simulink model "EAF_simscape"  (R2025b)
settings: Solver=ode23t  StartTime=0.0  StopTime=5  RelTol=1e-3
undefined symbols (not defined in the file or in its folder): Three_PhaseSeriesRLCLoad_class, Three_PhaseSource_class, Three_PhaseTransformer_2_class, Three_PhaseTransformer_T_class, Three_PhaseV_IMeasuremen_class
libraries: ee_lib x12, nesl_utility x9, fl_lib x6, elec_conv_Three_PhaseV_IMeasuremen x4, eeRmsMeasurement x3, elec_conv_sl_RMS x3, spsVariableResistorLib x3, elec_conv_Three_PhaseSeriesRLCBran x3, elec_conv_Three_PhaseSeriesRLCLoad x2, elec_conv_Three_PhaseTransformer_2 x2, elec_conv_Three_PhaseTransformer_T x1, elec_conv_Three_PhaseSource x1
(part 1 of 2)
settings Model: Creator=LYG  LastModifiedBy=LYG
settings DebuggingCC: SaveWithParameterizedLinksMsg=none

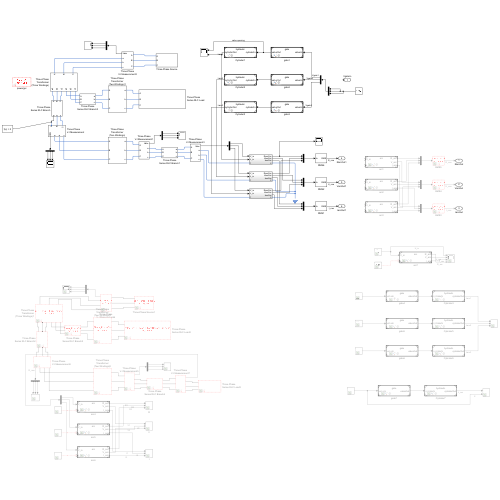
[thumbnail: Simulink's stored preview of the top-level diagram]
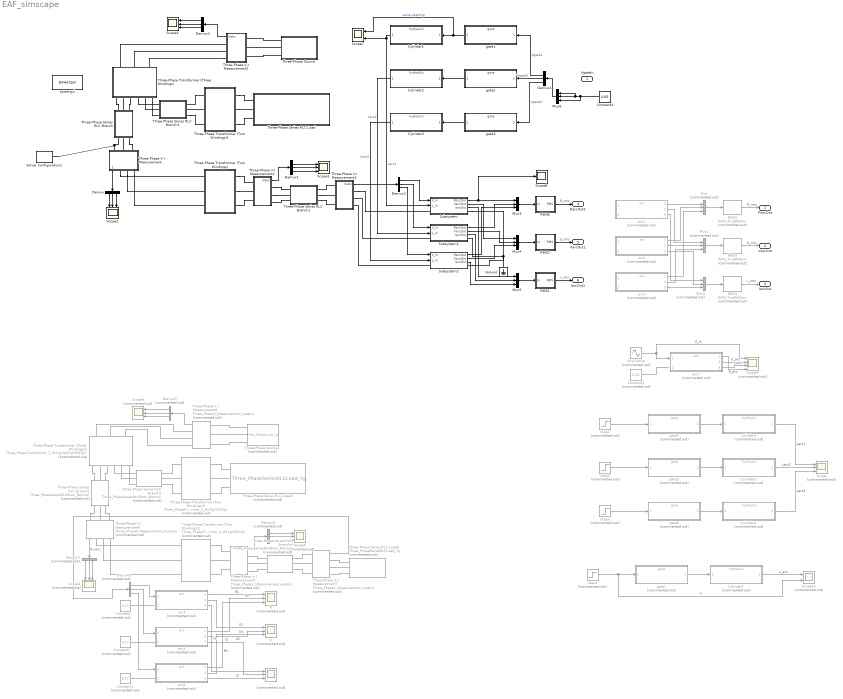
== system EAF_simscape ==
  VgateIn : Inport
  Constant : Constant  Commented=on  Value=0.17
  Constant1 : Constant  Commented=on  Value=0.17
  Constant2 : Constant  Commented=on  Value=0.17
  Constant3 : Constant  Commented=on  Value=0.15
  Constant4 : Constant  Value=0.65
  Cylinder1 : ModelReference  ModelNameDialog=hydraulic.slx  UsingDefaultArgumentValue=0,0,0,0,0,0,0,0,0  SimulationMode=Normal  ModelReferenceVersion=1.17  Ap=0.0314  Ct=2.4e-12  Fforce=90000  Gmass=9000  Kc=1.68e-9  Kq=1.63  Ve=0.11304  beta_e=7e8  L_init=0.15
  Cylinder2 : ModelReference  ModelNameDialog=hydraulic.slx  UsingDefaultArgumentValue=0,0,0,0,0,0,0,0,0  SimulationMode=Normal  ModelReferenceVersion=1.17  Ap=0.0314  Ct=2.4e-12  Fforce=90000  Gmass=9000  Kc=1.68e-9  Kq=1.63  Ve=0.11304  beta_e=7e8  L_init=0.15
  Cylinder3 : ModelReference  ModelNameDialog=hydraulic.slx  UsingDefaultArgumentValue=0,0,0,0,0,0,0,0,0  SimulationMode=Normal  ModelReferenceVersion=1.17  Ap=0.0314  Ct=2.4e-12  Fforce=90000  Gmass=9000  Kc=1.68e-9  Kq=1.63  Ve=0.11304  beta_e=7e8  L_init=0.15
  Cylinder4 : ModelReference  Commented=on  ModelNameDialog=hydraulic.slx  UsingDefaultArgumentValue=0,0,0,0,0,0,0,0,0  SimulationMode=Normal  ModelReferenceVersion=1.17  Ap=0.0314  Ct=2.4e-12  Fforce=90000  Gmass=9000  Kc=1.68e-9  Kq=1.63  Ve=0.11304  beta_e=7e8  L_init=15
  Cylinder5 : ModelReference  Commented=on  ModelNameDialog=hydraulic.slx  UsingDefaultArgumentValue=0,0,0,0,0,0,0,0,0  SimulationMode=Normal  ModelReferenceVersion=1.17  Ap=0.0314  Ct=2.4e-12  Fforce=90000  Gmass=9000  Kc=1.68e-9  Kq=1.63  Ve=0.11304  beta_e=7e8  L_init=15
  Cylinder6 : ModelReference  Commented=on  ModelNameDialog=hydraulic.slx  UsingDefaultArgumentValue=0,0,0,0,0,0,0,0,0  SimulationMode=Normal  ModelReferenceVersion=1.17  Ap=0.0314  Ct=2.4e-12  Fforce=90000  Gmass=9000  Kc=1.68e-9  Kq=1.63  Ve=0.11304  beta_e=7e8  L_init=15
  Cylinder7 : ModelReference  Commented=on  ModelNameDialog=hydraulic.slx  UsingDefaultArgumentValue=0,0,0,0,0,0,0,0,0  SimulationMode=Normal  ModelReferenceVersion=1.17  Ap=0.0314  Ct=2.4e-12  Fforce=90000  Gmass=9000  Kc=1.68e-9  Kq=1.63  Ve=0.11304  beta_e=7e8  L_init=0.5
  Demux{,1..4} (5 alike) : Demux  Outputs=3
  Demux{5..8} (4 alike) : Demux  Commented=on  Outputs=3
  Ground : fl_lib/Electrical/Electrical Elements/Electrical Reference
  I : Scope  Commented=on  NumInputPorts=3
      settings: ActiveDisplayYMinimum=-181487.67004  ActiveDisplayYMaximum=204820.87282  DataLoggingVariableName=ScopeData4
  Mux : Mux  Commented=on  Inputs=3
  Mux1 : Mux  Commented=on  Inputs=3
  Mux2 : Mux  Commented=on  Inputs=3
  Mux{3..6} (4 alike) : Mux  Inputs=3
  R : Scope  Commented=on  NumInputPorts=3
      settings: ActiveDisplayYMinimum=-0.00531  ActiveDisplayYMaximum=0.04981  DataLoggingVariableName=ScopeData5
  RMS1 : Subsystem
      settings: OpenFcn=elec.conv.unmask(gcb);
  RMS2 : Subsystem
      settings: OpenFcn=elec.conv.unmask(gcb);
  RMS3 : elec_conv_sl_RMS/RMS_TrueRMSon  Commented=on  SystemSampleTime=-1  VariantActivationTime=update diagram  EmptyChoice=off  PassThrough=off  PassThroughVariantControl=(default)  EmptyChoiceVariantControl=(default)  AllowFlexibleInterface=on  Latency=0  AutoFrameSizeCalculation=off
  RMS4 : elec_conv_sl_RMS/RMS_TrueRMSon  Commented=on  SystemSampleTime=-1  VariantActivationTime=update diagram  EmptyChoice=off  PassThrough=off  PassThroughVariantControl=(default)  EmptyChoiceVariantControl=(default)  AllowFlexibleInterface=on  Latency=0  AutoFrameSizeCalculation=off
  RMS5 : elec_conv_sl_RMS/RMS_TrueRMSon  Commented=on  SystemSampleTime=-1  VariantActivationTime=update diagram  EmptyChoice=off  PassThrough=off  PassThroughVariantControl=(default)  EmptyChoiceVariantControl=(default)  AllowFlexibleInterface=on  Latency=0  AutoFrameSizeCalculation=off
  RMS6 : Subsystem
      settings: OpenFcn=elec.conv.unmask(gcb);
  Scope{,1,5..6} (4 alike) : Scope  Commented=on  NumInputPorts=3
      Scope settings: ActiveDisplayYMinimum=13.76369  ActiveDisplayYMaximum=16.01617  DataLoggingVariableName=ScopeData4
      Scope1 settings: ActiveDisplayYMinimum=-4346.80314  ActiveDisplayYMaximum=39121.22823
      Scope5 settings: ActiveDisplayYMinimum=-7403.31219  ActiveDisplayYMaximum=7403.31279  DataLoggingVariableName=ScopeData2
      Scope6 settings: ActiveDisplayYMinimum=-194335.71856  ActiveDisplayYMaximum=194335.71856  DataLoggingVariableName=ScopeData3
  Scope10 : Scope  Commented=on  NumInputPorts=2
      settings: ActiveDisplayYMinimum=0.16708  ActiveDisplayYMaximum=1.06427  DataLoggingVariableName=ScopeData2
  Scope2 : Scope  NumInputPorts=3
      settings: ActiveDisplayYMinimum=-54351.26141  ActiveDisplayYMaximum=61130.65536
  Scope3 : Scope  NumInputPorts=3
      settings: ActiveDisplayYMinimum=-666.22173  ActiveDisplayYMaximum=595.66342  DataLoggingVariableName=ScopeData2
  Scope4 : Scope  NumInputPorts=3
      settings: ActiveDisplayYMinimum=-194453.93834  ActiveDisplayYMaximum=194453.93834  DataLoggingVariableName=ScopeData3
  Scope7 : Scope  NumInputPorts=2
      settings: ActiveDisplayYMinimum=-0.00342  ActiveDisplayYMaximum=0.00705
  Scope8 : Scope
      settings: ActiveDisplayYMinimum=-66.36555  ActiveDisplayYMaximum=597.29198
  Scope9 : Scope  Commented=on  NumInputPorts=4
      settings: ActiveDisplayYMinimum=-429.56648  ActiveDisplayYMaximum=429.56274
  Sine Wave : Sin  Commented=on  Amplitude=sqrt(2) * 243  Frequency=2 * pi * 60  SampleTime=0
  Solver Configuration1 : nesl_utility/Solver Configuration  PhysicalDomain=network_engine_domain  SubClassName=solver  LeftPortType=input  RightPortType=generic  Tones=[]  Harmonics=[]  SimulateNoise=off  Profile=off  UseLocalSampling=off  EnableSwitchedLinearOptims=on  FrequencyDomain=off  UseCCode=off  RelTol=0.001  AbsTol=0.001  MinStep=1e-09  ToWorkspace=off  RevertToSquareIcSolve=off  NumHomotopyIterations=100  PhasorMode=off  PhasorModeNumHarmonics=1  ConsistencySolver=NEWTON_XTOL_AFTER_FTOL  IndexReductionMethod=DerivativeReplacement  DoDC=off  ResidualTolerance=1e-09  ConsistencyTolSource=GLOBAL  ConsistencyAbsTol=0.001  ConsistencyRelTol=0.001  ConsistencyTolFactor=0.001  UseLocalSolver=off  LocalSolverChoice=NE_BACKWARD_EULER_ADVANCER  ResolveIndetEquations=on  FunctionEvalNumThread=1  LocalSolverSampleTime=0.001  DoFixedCost=off  MaxNonlinIter=3  MaxModeIter=2  ComputeImpulses=off  ImpulseIterations=2  LinearAlgebra=auto  LinearAlgebraNumThread=0  EquationFormulation=NE_TIME_EF  DelaysMemoryBudget=1024  AutomaticFiltering=on  FilteringTimeConstant=0.001  PartitionStorageMethod=AS_NEEDED  PartitionMemoryBudget=1024  PartitionMethod=ROBUST  MultibodyUseLocalSolver=off  MultibodyLocalSolverChoice=ODE1  MultibodyLocalSolverSampleTime=0.001
  Step1 : Step  Commented=on  Time=5  After=5  SampleTime=0
  Step2 : Step  Commented=on  Time=5  Before=5  After=0  SampleTime=0
  Step3 : Step  Commented=on  Time=3  Before=5  After=-5  SampleTime=0
  Step4 : Step  Commented=on  Time=3  Before=5  After=-5  SampleTime=0
  Subsystem : Subsystem
  Subsystem1 : Subsystem
  Subsystem2 : Subsystem
  Three-Phase Series RLC Branch : Subsystem
      settings: AttributesFormatString=\n  OpenFcn=elec.conv.unmask(gcb);
  Three-Phase Series RLC Branch1 : Subsystem
      settings: AttributesFormatString=\n  OpenFcn=elec.conv.unmask(gcb);
  Three-Phase Series RLC Branch2 : elec_conv_Three_PhaseSeriesRLCBran/Three_PhaseSeriesRLCBran_Normal  Commented=on  component_structure=1  R=0.256  L=0.001  C=1e-06
      settings: AttributesFormatString=\n
  Three-Phase Series RLC Branch3 : Subsystem
      settings: AttributesFormatString=\n  OpenFcn=elec.conv.unmask(gcb);
  Three-Phase Series RLC Branch4 : elec_conv_Three_PhaseSeriesRLCBran/Three_PhaseSeriesRLCBran_Normal  Commented=on  component_structure=4  R=0.0004  L=1.115e-05  C=1e-06
      settings: AttributesFormatString=\n
  Three-Phase Series RLC Branch5 : elec_conv_Three_PhaseSeriesRLCBran/Three_PhaseSeriesRLCBran_Normal  Commented=on  component_structure=1  R=0.256  L=0.001  C=1e-06
      settings: AttributesFormatString=\n
  Three-Phase Series RLC Load : Subsystem
      settings: AttributesFormatString=\n  OpenFcn=elec.conv.unmask(gcb);
  Three-Phase Series RLC Load2 : elec_conv_Three_PhaseSeriesRLCLoad/Three_PhaseSeriesRLCLoad_Yg  Commented=on  VRated=1000  Vmag0=1000  FRated=60  P=10000  Qpos=100  Qneg=Three_PhaseSeriesRLCLoad_class(100).objParamMappingDerived.NewDerivedParam.Qneg  component_structure_PQ=7  component_structure=7
      settings: AttributesFormatString=\n
  Three-Phase Series RLC Load3 : elec_conv_Three_PhaseSeriesRLCLoad/Three_PhaseSeriesRLCLoad_Yg  Commented=on  VRated=1000  Vmag0=1000  FRated=60  P=10000  Qpos=100  Qneg=Three_PhaseSeriesRLCLoad_class(100).objParamMappingDerived.NewDerivedParam.Qneg  component_structure_PQ=7  component_structure=7
      settings: AttributesFormatString=\n
  Three-Phase Transformer (Three Windings) : Subsystem
      settings: OpenFcn=elec.conv.unmask(gcb);
  Three-Phase Transformer (Three Windings)1 : elec_conv_Three_PhaseTransformer_T/Three_PhaseTransformer_T_W1YgYW2YgYW3YgY  Commented=on  SRated=250000000  FRated=60  VRated1=110000  VRated2=35000  VRated3=35000  phi_specify=off  phi_priority=None  pu_Rw1=Three_PhaseTransformer_T_class('Yg','Yg','Yg','pu',[250000000 60],[110000 1.186 0.08],[35000 0.256 0.08],[35000 0.002 0.08],499.98,500,0.5,[0 0;0.0024 1.2;1 1.52],[0.8 -0.8 0.69999],'off','off').objParamMappingDerived.NewDerivedParam.pu_Rw1  pu_Xl1=Three_PhaseTransformer_T_class('Yg','Yg','Yg','pu',[250000000 60],[110000 1.186 0.08],[35000 0.256 0.08],[35000 0.002 0.08],499.98,500,0.5,[0 0;0.0024 1.2;1 1.52],[0.8 -0.8 0.69999],'off','off').objParamMappingDerived.NewDerivedParam.pu_Xl1  pu_Rw2=Three_PhaseTransformer_T_class('Yg','Yg','Yg','pu',[250000000 60],[110000 1.186 0.08],[35000 0.256 0.08],[35000 0.002 0.08],499.98,500,0.5,[0 0;0.0024 1.2;1 1.52],[0.8 -0.8 0.69999],'off','off').objParamMappingDerived.NewDerivedParam.pu_Rw2  pu_Xl2=Three_PhaseTransformer_T_class('Yg','Yg','Yg','pu',[250000000 60],[110000 1.186 0.08],[35000 0.256 0.08],[35000 0.002 0.08],499.98,500,0.5,[0 0;0.0024 1.2;1 1.52],[0.8 -0.8 0.69999],'off','off').objParamMappingDerived.NewDerivedParam.pu_Xl2  pu_Rw3=Three_PhaseTransformer_T_class('Yg','Yg','Yg','pu',[250000000 60],[110000 1.186 0.08],[35000 0.256 0.08],[35000 0.002 0.08],499.98,500,0.5,[0 0;0.0024 1.2;1 1.52],[0.8 -0.8 0.69999],'off','off').objParamMappingDerived.NewDerivedParam.pu_Rw3  pu_Xl3=Three_PhaseTransformer_T_class('Yg','Yg','Yg','pu',[250000000 60],[110000 1.186 0.08],[35000 0.256 0.08],[35000 0.002 0.08],499.98,500,0.5,[0 0;0.0024 1.2;1 1.52],[0.8 -0.8 0.69999],'off','off').objParamMappingDerived.NewDerivedParam.pu_Xl3  pu_Rm=Three_PhaseTransformer_T_class('Yg','Yg','Yg','pu',[250000000 60],[110000 1.186 0.08],[35000 0.256 0.08],[35000 0.002 0.08],499.98,500,0.5,[0 0;0.0024 1.2;1 1.52],[0.8 -0.8 0.69999],'off','off').objParamMappingDerived.NewDerivedParam.pu_Rm  pu_Xm=Three_PhaseTransformer_T_class('Yg','Yg','Yg','pu',[250000000 60],[110000 1.186 0.08],[35000 0.256 0.08],[35000 0.002 0.08],499.98,500,0.5,[0 0;0.0024 1.2;1 1.52],[0.8 -0.8 0.69999],'off','off').objParamMappingDerived.NewDerivedParam.pu_Xm  pu_X0=Three_PhaseTransformer_T_class('Yg','Yg','Yg','pu',[250000000 60],[110000 1.186 0.08],[35000 0.256 0.08],[35000 0.002 0.08],499.98,500,0.5,[0 0;0.0024 1.2;1 1.52],[0.8 -0.8 0.69999],'off','off').objParamMappingDerived.NewDerivedParam.pu_X0  current_data=Three_PhaseTransformer_T_class('Yg','Yg','Yg','pu',[250000000 60],[110000 1.186 0.08],[35000 0.256 0.08],[35000 0.002 0.08],499.98,500,0.5,[0 0;0.0024 1.2;1 1.52],[0.8 -0.8 0.69999],'off','off').objParamMappingDerived.NewDerivedParam.current_data  magnetic_flux_data=Three_PhaseTransformer_T_class('Yg','Yg','Yg','pu',[250000000 60],[110000 1.186 0.08],[35000 0.256 0.08],[35000 0.002 0.08],499.98,500,0.5,[0 0;0.0024 1.2;1 1.52],[0.8 -0.8 0.69999],'off','off').objParamMappingDerived.NewDerivedParam.magnetic_flux_data  phi=Three_PhaseTransformer_T_class('Yg','Yg','Yg','pu',[250000000 60],[110000 1.186 0.08],[35000 0.256 0.08],[35000 0.002 0.08],499.98,500,0.5,[0 0;0.0024 1.2;1 1.52],[0.8 -0.8 0.69999],'off','off').objParamMappingDerived.NewDerivedParam.phi  Winding1Connection=3  Winding2Connection=3  Winding3Connection=3  saturation_option=1  CoreType=2
  Three-Phase Transformer (Two Windings) : Subsystem
      settings: OpenFcn=elec.conv.unmask(gcb);
  Three-Phase Transformer (Two Windings)1 : Subsystem
      settings: OpenFcn=elec.conv.unmask(gcb);
  Three-Phase Transformer (Two Windings)2 : elec_conv_Three_PhaseTransformer_2/Three_PhaseTransformer_2_W1YgYW2YgY  Commented=on  SRated=250000000  FRated=60  VRated1=35000  VRated2=440.02  phi_specify=off  phi_priority=None  pu_Rw1=Three_PhaseTransformer_2_class('Yg','Yg','pu',[250000000 60],[35000 6.9e-05 2.2e-06],[440.02 6.9e-05 2.2e-06],500,500,0.5,[0 0;0.0024 1.2;1 1.52],[0.8 -0.8 0.7],'off','off').objParamMappingDerived.NewDerivedParam.pu_Rw1  pu_Xl1=Three_PhaseTransformer_2_class('Yg','Yg','pu',[250000000 60],[35000 6.9e-05 2.2e-06],[440.02 6.9e-05 2.2e-06],500,500,0.5,[0 0;0.0024 1.2;1 1.52],[0.8 -0.8 0.7],'off','off').objParamMappingDerived.NewDerivedParam.pu_Xl1  pu_Rw2=Three_PhaseTransformer_2_class('Yg','Yg','pu',[250000000 60],[35000 6.9e-05 2.2e-06],[440.02 6.9e-05 2.2e-06],500,500,0.5,[0 0;0.0024 1.2;1 1.52],[0.8 -0.8 0.7],'off','off').objParamMappingDerived.NewDerivedParam.pu_Rw2  pu_Xl2=Three_PhaseTransformer_2_class('Yg','Yg','pu',[250000000 60],[35000 6.9e-05 2.2e-06],[440.02 6.9e-05 2.2e-06],500,500,0.5,[0 0;0.0024 1.2;1 1.52],[0.8 -0.8 0.7],'off','off').objParamMappingDerived.NewDerivedParam.pu_Xl2  pu_Rm=Three_PhaseTransformer_2_class('Yg','Yg','pu',[250000000 60],[35000 6.9e-05 2.2e-06],[440.02 6.9e-05 2.2e-06],500,500,0.5,[0 0;0.0024 1.2;1 1.52],[0.8 -0.8 0.7],'off','off').objParamMappingDerived.NewDerivedParam.pu_Rm  pu_Xm=Three_PhaseTransformer_2_class('Yg','Yg','pu',[250000000 60],[35000 6.9e-05 2.2e-06],[440.02 6.9e-05 2.2e-06],500,500,0.5,[0 0;0.0024 1.2;1 1.52],[0.8 -0.8 0.7],'off','off').objParamMappingDerived.NewDerivedParam.pu_Xm  pu_X0=Three_PhaseTransformer_2_class('Yg','Yg','pu',[250000000 60],[35000 6.9e-05 2.2e-06],[440.02 6.9e-05 2.2e-06],500,500,0.5,[0 0;0.0024 1.2;1 1.52],[0.8 -0.8 0.7],'off','off').objParamMappingDerived.NewDerivedParam.pu_X0  current_data=Three_PhaseTransformer_2_class('Yg','Yg','pu',[250000000 60],[35000 6.9e-05 2.2e-06],[440.02 6.9e-05 2.2e-06],500,500,0.5,[0 0;0.0024 1.2;1 1.52],[0.8 -0.8 0.7],'off','off').objParamMappingDerived.NewDerivedParam.current_data  magnetic_flux_data=Three_PhaseTransformer_2_class('Yg','Yg','pu',[250000000 60],[35000 6.9e-05 2.2e-06],[440.02 6.9e-05 2.2e-06],500,500,0.5,[0 0;0.0024 1.2;1 1.52],[0.8 -0.8 0.7],'off','off').objParamMappingDerived.NewDerivedParam.magnetic_flux_data  phi=Three_PhaseTransformer_2_class('Yg','Yg','pu',[250000000 60],[35000 6.9e-05 2.2e-06],[440.02 6.9e-05 2.2e-06],500,500,0.5,[0 0;0.0024 1.2;1 1.52],[0.8 -0.8 0.7],'off','off').objParamMappingDerived.NewDerivedParam.phi  Winding1Connection=3  Winding2Connection=3  saturation_option=1  CoreType=2
  Three-Phase Transformer (Two Windings)3 : elec_conv_Three_PhaseTransformer_2/Three_PhaseTransformer_2_W1YgYW2YgY  Commented=on  SRated=250000000  FRated=60  VRated1=735000  VRated2=8820  phi_specify=off  phi_priority=None  pu_Rw1=Three_PhaseTransformer_2_class('Yg','Yg','pu',[250000000 60],[735000 6.9e-05 2.2e-06],[8820 6.9e-05 2.2e-06],500,500,0.5,[0 0;0.0024 1.2;1 1.52],[0.8 -0.8 0.7],'off','off').objParamMappingDerived.NewDerivedParam.pu_Rw1  pu_Xl1=Three_PhaseTransformer_2_class('Yg','Yg','pu',[250000000 60],[735000 6.9e-05 2.2e-06],[8820 6.9e-05 2.2e-06],500,500,0.5,[0 0;0.0024 1.2;1 1.52],[0.8 -0.8 0.7],'off','off').objParamMappingDerived.NewDerivedParam.pu_Xl1  pu_Rw2=Three_PhaseTransformer_2_class('Yg','Yg','pu',[250000000 60],[735000 6.9e-05 2.2e-06],[8820 6.9e-05 2.2e-06],500,500,0.5,[0 0;0.0024 1.2;1 1.52],[0.8 -0.8 0.7],'off','off').objParamMappingDerived.NewDerivedParam.pu_Rw2  pu_Xl2=Three_PhaseTransformer_2_class('Yg','Yg','pu',[250000000 60],[735000 6.9e-05 2.2e-06],[8820 6.9e-05 2.2e-06],500,500,0.5,[0 0;0.0024 1.2;1 1.52],[0.8 -0.8 0.7],'off','off').objParamMappingDerived.NewDerivedParam.pu_Xl2  pu_Rm=Three_PhaseTransformer_2_class('Yg','Yg','pu',[250000000 60],[735000 6.9e-05 2.2e-06],[8820 6.9e-05 2.2e-06],500,500,0.5,[0 0;0.0024 1.2;1 1.52],[0.8 -0.8 0.7],'off','off').objParamMappingDerived.NewDerivedParam.pu_Rm  pu_Xm=Three_PhaseTransformer_2_class('Yg','Yg','pu',[250000000 60],[735000 6.9e-05 2.2e-06],[8820 6.9e-05 2.2e-06],500,500,0.5,[0 0;0.0024 1.2;1 1.52],[0.8 -0.8 0.7],'off','off').objParamMappingDerived.NewDerivedParam.pu_Xm  pu_X0=Three_PhaseTransformer_2_class('Yg','Yg','pu',[250000000 60],[735000 6.9e-05 2.2e-06],[8820 6.9e-05 2.2e-06],500,500,0.5,[0 0;0.0024 1.2;1 1.52],[0.8 -0.8 0.7],'off','off').objParamMappingDerived.NewDerivedParam.pu_X0  current_data=Three_PhaseTransformer_2_class('Yg','Yg','pu',[250000000 60],[735000 6.9e-05 2.2e-06],[8820 6.9e-05 2.2e-06],500,500,0.5,[0 0;0.0024 1.2;1 1.52],[0.8 -0.8 0.7],'off','off').objParamMappingDerived.NewDerivedParam.current_data  magnetic_flux_data=Three_PhaseTransformer_2_class('Yg','Yg','pu',[250000000 60],[735000 6.9e-05 2.2e-06],[8820 6.9e-05 2.2e-06],500,500,0.5,[0 0;0.0024 1.2;1 1.52],[0.8 -0.8 0.7],'off','off').objParamMappingDerived.NewDerivedParam.magnetic_flux_data  phi=Three_PhaseTransformer_2_class('Yg','Yg','pu',[250000000 60],[735000 6.9e-05 2.2e-06],[8820 6.9e-05 2.2e-06],500,500,0.5,[0 0;0.0024 1.2;1 1.52],[0.8 -0.8 0.7],'off','off').objParamMappingDerived.NewDerivedParam.phi  Winding1Connection=3  Winding2Connection=3  saturation_option=1  CoreType=2
  Three-Phase V-I Measurement : Subsystem
      settings: OpenFcn=elec.conv.unmask(gcb);
  Three-Phase V-I Measurement1 : Subsystem
      settings: OpenFcn=elec.conv.unmask(gcb);
  Three-Phase V-I Measurement2 : Subsystem
      settings: OpenFcn=elec.conv.unmask(gcb);
  Three-Phase V-I Measurement3 : Subsystem
      settings: OpenFcn=elec.conv.unmask(gcb);
  Three-Phase V-I Measurement{4..7} (4 alike) : elec_conv_Three_PhaseV_IMeasuremen/Three_PhaseV_IMeasuremen_VyesIno  Commented=on  SRated=100000000  VRated=500000  vMeasurementType=1  outputUnit=2  GotoTagI=Iabc  GotoTagV=Vabc  IG=Three_PhaseV_IMeasuremen_class('phase-to-phase','no','off','off','off',100000000,500000).objParamMappingDerived.NewDerivedParam.IG  VG=Three_PhaseV_IMeasuremen_class('phase-to-phase','no','off','off','off',100000000,500000).objParamMappingDerived.NewDerivedParam.VG
  Three-Phase Source : Subsystem
      settings: OpenFcn=elec.conv.unmask(gcb);
  Three-Phase Source1 : elec_conv_Three_PhaseSource/Three_PhaseSource_Yg  Commented=on  vline_rms=110000  shift=0  freq=60  SShortCircuit=100000000  XR=7  R=Three_PhaseSource_class(110000,60,1.186,0.01658,100000000,110000,7,'on','off').objParamMappingDerived.NewDerivedParam.R  L=Three_PhaseSource_class(110000,60,1.186,0.01658,100000000,110000,7,'on','off').objParamMappingDerived.NewDerivedParam.L  impedance_option=4
  V : Scope  Commented=on  NumInputPorts=3
      settings: ActiveDisplayYMinimum=-330.37837  ActiveDisplayYMaximum=329.45455
  arc{1..7} (7 alike) : ModelReference  Commented=on  ModelNameDialog=arc.slx  UsingDefaultArgumentValue=0,0,0,0,0,0,0  SimulationMode=Normal  ModelReferenceVersion=1.20  K1=221320  K2=0.00072  lambda=2  Xd=3e-3  rd=0.4e-3  f=50  U_PhaseRMS=243
  gate1 : ModelReference  ModelNameDialog=gate.slx  UsingDefaultArgumentValue=0,0,0,0,0,0,0  SimulationMode=Normal  ModelReferenceVersion=1.12  Ksvr=0.04  Ksvl=0.0276  Xmax=0.006  Xmin=-0.004  dl=-0.014  dr=0.014  k=0.15
  gate2 : ModelReference  ModelNameDialog=gate.slx  UsingDefaultArgumentValue=0,0,0,0,0,0,0  SimulationMode=Normal  ModelReferenceVersion=1.12  Ksvr=0.04  Ksvl=0.0276  Xmax=0.006  Xmin=-0.004  dl=-0.014  dr=0.014  k=0.15
  gate3 : ModelReference  ModelNameDialog=gate.slx  UsingDefaultArgumentValue=0,0,0,0,0,0,0  SimulationMode=Normal  ModelReferenceVersion=1.12  Ksvr=0.04  Ksvl=0.0276  Xmax=0.006  Xmin=-0.004  dl=-0.014  dr=0.014  k=0.15
  gate{4..7} (4 alike) : ModelReference  Commented=on  ModelNameDialog=gate.slx  UsingDefaultArgumentValue=0,0,0,0,0,0,0  SimulationMode=Normal  ModelReferenceVersion=1.12  Ksvr=0.04  Ksvl=0.0276  Xmax=0.006  Xmin=-0.004  dl=-0.014  dr=0.014  k=0.15
  powergui : sps_lib/powergui  Priority=1  SimulationMode=Discrete  SampleTime=5e-5  frequency=60  Iterations=50  frequencyindice=60  Pbase=100e6  ErrMax=1e-4  UnitsV=kV  UnitsW=MW  buscounter=0  FunctionMessages=off  echomessages=off  EnableUseOfTLC=off  CurrentSourceSwitches=off  DisableSnubberDevices=off  DisableRonSwitches=off  DisableVfSwitches=off  DisplayEquations=off  AutomaticDiscreteSolvers=off  SolverType=Tustin/Backward Euler (TBE)  Interpol=off  ExternalGateDelay=off  methode=off  Ts=100  x0status=blocks  SPID=on  SwTol=0  HookPort=off  NonlinearTolerance=1e-4  nMaxIteration=100  ContinueOnMaxIteration=off  RestoreLinks=warning  ResistiveCurrentMeasurement=off  Frange=[0:2:500]  Ylog=off  Xlog=on  ShowGrid=off  save=off  variable=ZData  structure=0  ZoomFFT=off  StartTime=0.0  cycles=1  DisplayStyle=1  fundamental=60  FreqAxis=off  MaxFrequency=1000  frequencyindicesteady=1  RmsSteady=1  display=off
  RarcOut : Outport
  VarcOut : Outport  Port=2
  IarcOut : Outport  Port=3
  RarcOut1 : Outport  Port=4
  VarcOut1 : Outport  Port=5
  IarcOut1 : Outport  Port=6
  wires:
  Demux2/1 -> Scope4/1
  Demux2/3 -> Scope4/3
  Three-Phase V-I Measurement1/1(Vabc) -> Demux1/1
  Demux2/2 -> Scope4/2
  Demux1/3 -> Scope3/3
  Demux/2 -> Scope2/2
  Demux/1 -> Scope2/1
  Three-Phase V-I Measurement2/1(Vabc) -> Demux2/1
  Demux1/1 -> Scope3/1
  Three-Phase V-I Measurement/1(Vabc) -> Demux/1
  Demux/3 -> Scope2/3
  Demux1/2 -> Scope3/2
  gate2/1 -> Cylinder2/1
  gate1/1 -> Scope7/1, Cylinder1/1  "valve opening"
  gate3/1 -> Cylinder3/1
  Cylinder1/1 -> Subsystem/2(L_in), Scope7/2  "Larc1"
  Demux4/3 -> gate3/1  "Vgate3"
  Demux4/2 -> gate2/1  "Vgate2"
  Mux/1 -> RMS5/1
  Mux1/1 -> RMS4/1
  Mux2/1 -> RMS3/1
  arc1/1 -> Mux/1
  arc2/1 -> Mux/2
  arc3/1 -> Mux/3
  arc1/2 -> Mux1/1
  arc2/2 -> Mux1/2
  arc3/2 -> Mux1/3
  arc3/3 -> Mux2/3
  arc2/3 -> Mux2/2
  arc1/3 -> Mux2/1
  arc6/2 -> V/3  "V3"
  arc6/1 -> R/3  "R3"
  arc5/1 -> R/2  "R2"
  arc4/1 -> R/1  "R1"
  arc6/3 -> I/3  "I3"
  arc5/3 -> I/2  "I2"
  arc4/3 -> I/1  "I1"
  arc5/2 -> V/2  "V2"
  Demux8/2 -> arc5/1
  arc4/2 -> V/1  "V1"
  Three-Phase V-I Measurement7/1 -> Demux8/1
  Demux8/3 -> arc6/1
  Demux6/1 -> Scope5/1
  Demux6/2 -> Scope5/2
  Demux6/3 -> Scope5/3
  Demux8/1 -> arc4/1
  Three-Phase V-I Measurement5/1 -> Demux6/1
  Constant1/1 -> ?
  Constant2/1 -> ?
  gate6/1 -> Cylinder6/1
  gate5/1 -> Cylinder5/1
  gate4/1 -> Cylinder4/1
  Cylinder4/1 -> Scope/1  "Larc1"
  Cylinder5/1 -> Scope/2  "Larc2"
  Cylinder6/1 -> Scope/3  "Larc3"
  RMS3/1 -> IarcOut/1  "I_rms"
  RMS5/1 -> RarcOut/1  "R_rms"
  RMS4/1 -> VarcOut/1  "U_rms"
  Step1/1 -> gate4/1
  Step2/1 -> gate5/1
  Step3/1 -> gate6/1
  Demux5/2 -> Scope6/2
  Demux5/1 -> Scope6/1
  Demux5/3 -> Scope6/3
  Three-Phase V-I Measurement6/1 -> Demux5/1
  Three-Phase V-I Measurement4/1 -> Demux7/1  "R_rms"
  Demux7/1 -> Scope1/1
  Demux7/2 -> Scope1/2
  Demux7/3 -> Scope1/3
  Constant3/1 -> ?
  Sine Wave/1 -> Scope9/1, arc7/1  "U_in"
  arc7/2 -> Scope9/2  "U_arc"
  arc7/3 -> Scope9/3  "I_arc"
  arc7/1 -> Scope9/4  "R_arc"
  Constant/1 -> ?
  gate7/1 -> Cylinder7/1
  Step4/1 -> Scope10/2, gate7/1  "X"
  Cylinder7/1 -> Scope10/1  "L_arc"
  Demux3/1 -> Subsystem/1(V_in)
  Demux3/2 -> Subsystem1/1(V_in)
  Demux3/3 -> Subsystem2/1(V_in)
  Cylinder2/1 -> Subsystem1/2(L_in)  "Larc2"
  Cylinder3/1 -> Subsystem2/2(L_in)  "Larc3"
  RMS1/1(RMS) -> IarcOut1/1  "I_rms"
  Mux4/1 -> RMS2/1(In)
  Mux5/1 -> RMS1/1(In)
  Mux3/1 -> RMS6/1(In)
  RMS6/1(RMS) -> RarcOut1/1  "R_rms"
  RMS2/1(RMS) -> VarcOut1/1  "U_rms"
  Subsystem/1(RarcOut) -> Scope8/1, Mux3/1
  Subsystem1/1(RarcOut) -> Mux3/2
  Subsystem2/1(RarcOut) -> Mux3/3
  Subsystem/2(VarcOut) -> Mux4/1
  Subsystem1/2(VarcOut) -> Mux4/2
  Subsystem2/2(VarcOut) -> Mux4/3
  Subsystem/3(IarcOut) -> Mux5/1
  Subsystem1/3(IarcOut) -> Mux5/2
  Subsystem2/3(IarcOut) -> Mux5/3
  Three-Phase V-I Measurement3/1(Vabc) -> Demux3/1
  Demux4/1 -> gate1/1  "Vgate1"
  Constant4/1 -> Mux6/1, Mux6/2, Mux6/3
  Mux6/1 -> Demux4/1
  connections:
  Three-Phase Source/RConn2 -- Three-Phase V-I Measurement2/LConn2
  Three-Phase Transformer (Two Windings)/RConn3 -- Three-Phase V-I Measurement1/LConn3
  Three-Phase V-I Measurement1/RConn2 -- Three-Phase Series RLC Branch1/LConn2
  Three-Phase Transformer (Two Windings)/RConn1 -- Three-Phase V-I Measurement1/LConn1
  Three-Phase Series RLC Branch/RConn2 -- Three-Phase V-I Measurement/LConn2
  Three-Phase V-I Measurement2/RConn1 -- Three-Phase Transformer (Three Windings)/LConn1
  Three-Phase V-I Measurement1/RConn3 -- Three-Phase Series RLC Branch1/LConn3
  Three-Phase Transformer (Three Windings)/RConn2 -- Three-Phase Series RLC Branch/LConn2
  Three-Phase Transformer (Three Windings)/RConn1 -- Three-Phase Series RLC Branch/LConn1
  Three-Phase Transformer (Three Windings)/RConn3 -- Three-Phase Series RLC Branch/LConn3
  Three-Phase V-I Measurement2/RConn3 -- Three-Phase Transformer (Three Windings)/LConn3
  Three-Phase V-I Measurement/LConn1 -- Three-Phase Series RLC Branch/RConn1 -- Solver Configuration1/RConn1
  Three-Phase Source/RConn1 -- Three-Phase V-I Measurement2/LConn1
  Three-Phase Source/RConn3 -- Three-Phase V-I Measurement2/LConn3
  Three-Phase Series RLC Branch/RConn3 -- Three-Phase V-I Measurement/LConn3
  Three-Phase Transformer (Two Windings)/RConn2 -- Three-Phase V-I Measurement1/LConn2
  Three-Phase V-I Measurement1/RConn1 -- Three-Phase Series RLC Branch1/LConn1
  Three-Phase V-I Measurement2/RConn2 -- Three-Phase Transformer (Three Windings)/LConn2
  Three-Phase V-I Measurement3/LConn1 -- Three-Phase Series RLC Branch1/RConn1
  Three-Phase Series RLC Branch1/RConn2 -- Three-Phase V-I Measurement3/LConn2
  Three-Phase Series RLC Branch1/RConn3 -- Three-Phase V-I Measurement3/LConn3
  Three-Phase V-I Measurement/RConn2 -- Three-Phase Transformer (Two Windings)/LConn2
  Three-Phase V-I Measurement/RConn1 -- Three-Phase Transformer (Two Windings)/LConn1
  Three-Phase V-I Measurement/RConn3 -- Three-Phase Transformer (Two Windings)/LConn3
  Three-Phase Transformer (Two Windings)1/LConn1 -- Three-Phase Series RLC Branch3/RConn1
  Three-Phase Series RLC Branch3/RConn3 -- Three-Phase Transformer (Two Windings)1/LConn3
  Three-Phase Transformer (Two Windings)1/LConn2 -- Three-Phase Series RLC Branch3/RConn2
  Three-Phase Transformer (Three Windings)/RConn4 -- Three-Phase Series RLC Branch3/LConn1
  Three-Phase Transformer (Three Windings)/RConn5 -- Three-Phase Series RLC Branch3/LConn2
  Three-Phase Transformer (Three Windings)/RConn6 -- Three-Phase Series RLC Branch3/LConn3
  Three-Phase Transformer (Two Windings)1/RConn1 -- Three-Phase Series RLC Load/LConn1
  Three-Phase Transformer (Two Windings)1/RConn2 -- Three-Phase Series RLC Load/LConn2
  Three-Phase Transformer (Two Windings)1/RConn3 -- Three-Phase Series RLC Load/LConn3
  Three-Phase V-I Measurement5/RConn1 -- Three-Phase Series RLC Branch4/LConn1
  Three-Phase V-I Measurement7/RConn1 -- Three-Phase Series RLC Load3/LConn1
  Three-Phase Transformer (Two Windings)3/LConn1 -- Three-Phase Series RLC Branch5/RConn1
  Three-Phase Transformer (Two Windings)2/RConn1 -- Three-Phase V-I Measurement5/LConn1
  Three-Phase Transformer (Two Windings)3/LConn2 -- Three-Phase Series RLC Branch5/RConn2
  Three-Phase Transformer (Two Windings)3/RConn3 -- Three-Phase Series RLC Load2/LConn3
  Three-Phase Transformer (Two Windings)2/RConn2 -- Three-Phase V-I Measurement5/LConn2
  Three-Phase Transformer (Three Windings)1/RConn5 -- Three-Phase Series RLC Branch5/LConn2
  Three-Phase V-I Measurement4/RConn3 -- Three-Phase Transformer (Two Windings)2/LConn3
  Three-Phase V-I Measurement4/RConn1 -- Three-Phase Transformer (Two Windings)2/LConn1
  Three-Phase V-I Measurement7/RConn3 -- Three-Phase Series RLC Load3/LConn3
  Three-Phase Transformer (Three Windings)1/RConn3 -- Three-Phase Series RLC Branch2/LConn3
  Three-Phase Series RLC Branch5/RConn3 -- Three-Phase Transformer (Two Windings)3/LConn3
  Three-Phase Series RLC Branch4/RConn2 -- Three-Phase V-I Measurement7/LConn2
  Three-Phase Source1/RConn3 -- Three-Phase V-I Measurement6/LConn3
  Three-Phase Series RLC Branch4/RConn3 -- Three-Phase V-I Measurement7/LConn3
  Three-Phase V-I Measurement4/RConn2 -- Three-Phase Transformer (Two Windings)2/LConn2
  Three-Phase Transformer (Two Windings)3/RConn1 -- Three-Phase Series RLC Load2/LConn1
  Three-Phase V-I Measurement5/RConn3 -- Three-Phase Series RLC Branch4/LConn3
  Three-Phase Source1/RConn2 -- Three-Phase V-I Measurement6/LConn2
  Three-Phase Transformer (Two Windings)2/RConn3 -- Three-Phase V-I Measurement5/LConn3
  Three-Phase V-I Measurement6/RConn1 -- Three-Phase Transformer (Three Windings)1/LConn1
  Three-Phase V-I Measurement7/LConn1 -- Three-Phase Series RLC Branch4/RConn1
  Three-Phase Transformer (Three Windings)1/RConn1 -- Three-Phase Series RLC Branch2/LConn1
  Three-Phase Transformer (Three Windings)1/RConn2 -- Three-Phase Series RLC Branch2/LConn2
  Three-Phase V-I Measurement7/RConn2 -- Three-Phase Series RLC Load3/LConn2
  Three-Phase Source1/RConn1 -- Three-Phase V-I Measurement6/LConn1
  Three-Phase Transformer (Three Windings)1/RConn6 -- Three-Phase Series RLC Branch5/LConn3
  Three-Phase V-I Measurement6/RConn2 -- Three-Phase Transformer (Three Windings)1/LConn2
  Three-Phase Series RLC Branch2/RConn1 -- Three-Phase V-I Measurement4/LConn1
  Three-Phase Series RLC Branch2/RConn2 -- Three-Phase V-I Measurement4/LConn2
  Three-Phase Series RLC Branch2/RConn3 -- Three-Phase V-I Measurement4/LConn3
  Three-Phase V-I Measurement5/RConn2 -- Three-Phase Series RLC Branch4/LConn2
  Three-Phase Transformer (Three Windings)1/RConn4 -- Three-Phase Series RLC Branch5/LConn1
  Three-Phase Transformer (Two Windings)3/RConn2 -- Three-Phase Series RLC Load2/LConn2
  Three-Phase V-I Measurement6/RConn3 -- Three-Phase Transformer (Three Windings)1/LConn3
  Three-Phase V-I Measurement3/RConn1 -- Subsystem/LConn1
  Subsystem1/LConn1 -- Three-Phase V-I Measurement3/RConn2
  Subsystem2/LConn1 -- Three-Phase V-I Measurement3/RConn3
  Subsystem/RConn1 -- Subsystem1/RConn1 -- Subsystem2/RConn1 -- Ground/LConn1

== system EAF_simscape/RMS1 ==
  In : Inport
  RMS Measurement : eeRmsMeasurement/RMS Measurement  LabelModeActiveChoice=Total  F=60  SpecifyHarmonics=off  K=[0 1 2]  Ts=0
  RMS : Outport  VectorParamsAs1DForOutWhenUnconnected=off
  wires:
  RMS Measurement/1 -> RMS/1
  In/1 -> RMS Measurement/1

== system EAF_simscape/RMS2 ==
  In : Inport
  RMS Measurement : eeRmsMeasurement/RMS Measurement  LabelModeActiveChoice=Total  F=60  SpecifyHarmonics=off  K=[0 1 2]  Ts=0
  RMS : Outport  VectorParamsAs1DForOutWhenUnconnected=off
  wires:
  RMS Measurement/1 -> RMS/1
  In/1 -> RMS Measurement/1

== system EAF_simscape/RMS6 ==
  In : Inport
  RMS Measurement : eeRmsMeasurement/RMS Measurement  LabelModeActiveChoice=Total  F=60  SpecifyHarmonics=off  K=[0 1 2]  Ts=0
  RMS : Outport  VectorParamsAs1DForOutWhenUnconnected=off
  wires:
  RMS Measurement/1 -> RMS/1
  In/1 -> RMS Measurement/1

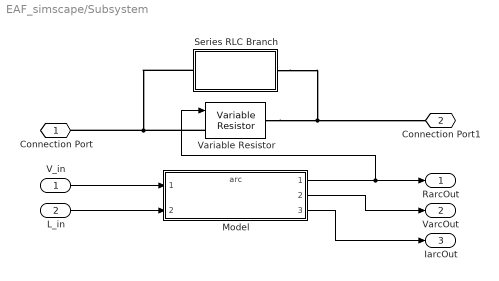
== system EAF_simscape/Subsystem ==
  V_in : Inport
  L_in : Inport  Port=2
  Model : ModelReference  ModelNameDialog=arc.slx  UsingDefaultArgumentValue=0,0,0,0,0,0,0  SimulationMode=Normal  ModelReferenceVersion=1.20  K1=221320  K2=0.00072  lambda=2  Xd=3e-3  rd=0.4e-3  f=50  U_PhaseRMS=243
  Series RLC Branch : Subsystem
      settings: OpenFcn=elec.conv.unmask(gcb);
  Variable Resistor : spsVariableResistorLib/Variable Resistor  Rabsmin=1e-3
      settings: LibrarySourceBlock=sps_lib/Passives/Variable Resistor
  Connection Port : PMIOPort  Side=Left
  Connection Port1 : PMIOPort  Port=2  Side=Right
  RarcOut : Outport
  VarcOut : Outport  Port=2
  IarcOut : Outport  Port=3
  wires:
  L_in/1 -> Model/2
  Model/1 -> Variable Resistor/1, RarcOut/1
  Model/2 -> VarcOut/1
  Model/3 -> IarcOut/1
  V_in/1 -> Model/1
  connections:
  Variable Resistor/LConn1 -- Series RLC Branch/LConn1 -- Connection Port/RConn1
  Variable Resistor/RConn1 -- Series RLC Branch/RConn1 -- Connection Port1/RConn1

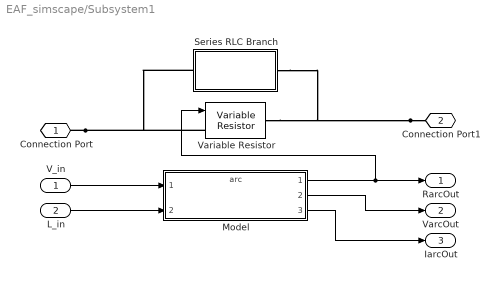
== system EAF_simscape/Subsystem1 ==
  V_in : Inport
  L_in : Inport  Port=2
  Model : ModelReference  ModelNameDialog=arc.slx  UsingDefaultArgumentValue=0,0,0,0,0,0,0  SimulationMode=Normal  ModelReferenceVersion=1.20  K1=221320  K2=0.00072  lambda=2  Xd=3e-3  rd=0.4e-3  f=50  U_PhaseRMS=243
  Series RLC Branch : Subsystem
      settings: OpenFcn=elec.conv.unmask(gcb);
  Variable Resistor : spsVariableResistorLib/Variable Resistor  Rabsmin=1e-3
  Connection Port : PMIOPort  Side=Left
  Connection Port1 : PMIOPort  Port=2  Side=Right
  RarcOut : Outport
  VarcOut : Outport  Port=2
  IarcOut : Outport  Port=3
  wires:
  L_in/1 -> Model/2
  Model/1 -> Variable Resistor/1, RarcOut/1
  Model/2 -> VarcOut/1
  Model/3 -> IarcOut/1
  V_in/1 -> Model/1
  connections:
  Connection Port/RConn1 -- Variable Resistor/LConn1 -- Series RLC Branch/LConn1
  Connection Port1/RConn1 -- Variable Resistor/RConn1 -- Series RLC Branch/RConn1

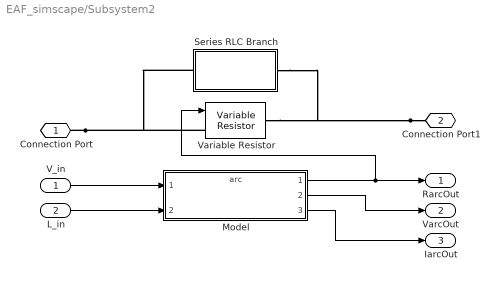
== system EAF_simscape/Subsystem2 ==
  V_in : Inport
  L_in : Inport  Port=2
  Model : ModelReference  ModelNameDialog=arc.slx  UsingDefaultArgumentValue=0,0,0,0,0,0,0  SimulationMode=Normal  ModelReferenceVersion=1.20  K1=221320  K2=0.00072  lambda=2  Xd=3e-3  rd=0.4e-3  f=50  U_PhaseRMS=243
  Series RLC Branch : Subsystem
      settings: OpenFcn=elec.conv.unmask(gcb);
  Variable Resistor : spsVariableResistorLib/Variable Resistor  Rabsmin=1e-3
  Connection Port : PMIOPort  Side=Left
  Connection Port1 : PMIOPort  Port=2  Side=Right
  RarcOut : Outport
  VarcOut : Outport  Port=2
  IarcOut : Outport  Port=3
  wires:
  L_in/1 -> Model/2
  Model/1 -> Variable Resistor/1, RarcOut/1
  Model/2 -> VarcOut/1
  Model/3 -> IarcOut/1
  V_in/1 -> Model/1
  connections:
  Connection Port/RConn1 -- Variable Resistor/LConn1 -- Series RLC Branch/LConn1
  Connection Port1/RConn1 -- Variable Resistor/RConn1 -- Series RLC Branch/RConn1

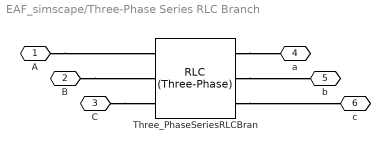
== system EAF_simscape/Three-Phase Series RLC Branch ==
  Three_PhaseSeriesRLCBran : ee_lib/Passive/RLC Assemblies/RLC (Three-Phase)  port_option=ee.enum.threePhasePort.expanded  component_structure=1  R=0.256 Ohm  L=0.001 H  C=1e-06 F  R_parasitic=1e-6 Ohm  G_parasitic=1e-6 1/Ohm  IL_specify=on  IL_priority=High  IL=[0, 0, 0] A  IL_nominal_specify=off  IL_nominal_value=1  IL_nominal_unit=A  VC_specify=on  VC_priority=High  VC=[0, 0, 0] V  VC_nominal_specify=off  VC_nominal_value=1  VC_nominal_unit=V
      settings: InternalSimscapePortConfiguration="{\"Bottom\":[],\"Left\":[{\"id\":\"a1\",\"label\":\"a1\",\"type\":\"foundation.electrical.electrical\"},{\"id\":\"b1\",\"label\":\"b1\",\"type\":\"foundation.electrical.electrical\"},{\"id\":\"c1\",\"label\":\"c1\",\"type\":\"foundation.electrical.electrical\"}],\"Right\":[{\"id\":\"a2\",\"label\":\"a2\",\"type\":\"foundation.electrical.electrical\"},{\"id\":\"b2\",\"label\":\"b2\",\"type\":\"foundation.electrical.electrical\"},{\"id\":\"c2\",\"label\":\"c2\",\"type\":\"foundation.electrical.electrical\"}],\"Top\":[]}"
  A : PMIOPort  Side=Left
  B : PMIOPort  Port=2  Side=Left
  C : PMIOPort  Port=3  Side=Left
  a : PMIOPort  Port=4  Side=Right
  b : PMIOPort  Port=5  Side=Right
  c : PMIOPort  Port=6  Side=Right
  connections:
  Three_PhaseSeriesRLCBran/RConn3 -- c/RConn1
  Three_PhaseSeriesRLCBran/RConn2 -- b/RConn1
  Three_PhaseSeriesRLCBran/RConn1 -- a/RConn1
  C/RConn1 -- Three_PhaseSeriesRLCBran/LConn3
  B/RConn1 -- Three_PhaseSeriesRLCBran/LConn2
  A/RConn1 -- Three_PhaseSeriesRLCBran/LConn1

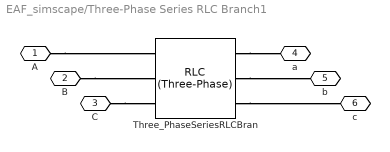
== system EAF_simscape/Three-Phase Series RLC Branch1 ==
  Three_PhaseSeriesRLCBran : ee_lib/Passive/RLC Assemblies/RLC (Three-Phase)  port_option=ee.enum.threePhasePort.expanded  component_structure=4  R=0.0004 Ohm  L=1.115e-05 H  C=1e-06 F  R_parasitic=1e-6 Ohm  G_parasitic=1e-6 1/Ohm  IL_specify=on  IL_priority=High  IL=[0, 0, 0] A  IL_nominal_specify=off  IL_nominal_value=1  IL_nominal_unit=A  VC_specify=on  VC_priority=High  VC=[0, 0, 0] V  VC_nominal_specify=off  VC_nominal_value=1  VC_nominal_unit=V
      settings: InternalSimscapePortConfiguration="{\"Bottom\":[],\"Left\":[{\"id\":\"a1\",\"label\":\"a1\",\"type\":\"foundation.electrical.electrical\"},{\"id\":\"b1\",\"label\":\"b1\",\"type\":\"foundation.electrical.electrical\"},{\"id\":\"c1\",\"label\":\"c1\",\"type\":\"foundation.electrical.electrical\"}],\"Right\":[{\"id\":\"a2\",\"label\":\"a2\",\"type\":\"foundation.electrical.electrical\"},{\"id\":\"b2\",\"label\":\"b2\",\"type\":\"foundation.electrical.electrical\"},{\"id\":\"c2\",\"label\":\"c2\",\"type\":\"foundation.electrical.electrical\"}],\"Top\":[]}"
  A : PMIOPort  Side=Left
  B : PMIOPort  Port=2  Side=Left
  C : PMIOPort  Port=3  Side=Left
  a : PMIOPort  Port=4  Side=Right
  b : PMIOPort  Port=5  Side=Right
  c : PMIOPort  Port=6  Side=Right
  connections:
  Three_PhaseSeriesRLCBran/RConn3 -- c/RConn1
  Three_PhaseSeriesRLCBran/RConn2 -- b/RConn1
  Three_PhaseSeriesRLCBran/RConn1 -- a/RConn1
  C/RConn1 -- Three_PhaseSeriesRLCBran/LConn3
  B/RConn1 -- Three_PhaseSeriesRLCBran/LConn2
  A/RConn1 -- Three_PhaseSeriesRLCBran/LConn1

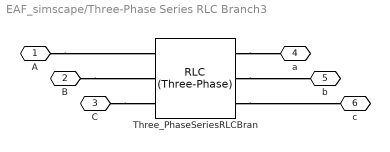
== system EAF_simscape/Three-Phase Series RLC Branch3 ==
  Three_PhaseSeriesRLCBran : ee_lib/Passive/RLC Assemblies/RLC (Three-Phase)  port_option=ee.enum.threePhasePort.expanded  component_structure=1  R=0.256 Ohm  L=0.001 H  C=1e-06 F  R_parasitic=1e-6 Ohm  G_parasitic=1e-6 1/Ohm  IL_specify=on  IL_priority=High  IL=[0, 0, 0] A  IL_nominal_specify=off  IL_nominal_value=1  IL_nominal_unit=A  VC_specify=on  VC_priority=High  VC=[0, 0, 0] V  VC_nominal_specify=off  VC_nominal_value=1  VC_nominal_unit=V
      settings: InternalSimscapePortConfiguration="{\"Bottom\":[],\"Left\":[{\"id\":\"a1\",\"label\":\"a1\",\"type\":\"foundation.electrical.electrical\"},{\"id\":\"b1\",\"label\":\"b1\",\"type\":\"foundation.electrical.electrical\"},{\"id\":\"c1\",\"label\":\"c1\",\"type\":\"foundation.electrical.electrical\"}],\"Right\":[{\"id\":\"a2\",\"label\":\"a2\",\"type\":\"foundation.electrical.electrical\"},{\"id\":\"b2\",\"label\":\"b2\",\"type\":\"foundation.electrical.electrical\"},{\"id\":\"c2\",\"label\":\"c2\",\"type\":\"foundation.electrical.electrical\"}],\"Top\":[]}"
  A : PMIOPort  Side=Left
  B : PMIOPort  Port=2  Side=Left
  C : PMIOPort  Port=3  Side=Left
  a : PMIOPort  Port=4  Side=Right
  b : PMIOPort  Port=5  Side=Right
  c : PMIOPort  Port=6  Side=Right
  connections:
  Three_PhaseSeriesRLCBran/RConn3 -- c/RConn1
  Three_PhaseSeriesRLCBran/RConn2 -- b/RConn1
  Three_PhaseSeriesRLCBran/RConn1 -- a/RConn1
  C/RConn1 -- Three_PhaseSeriesRLCBran/LConn3
  B/RConn1 -- Three_PhaseSeriesRLCBran/LConn2
  A/RConn1 -- Three_PhaseSeriesRLCBran/LConn1

== system EAF_simscape/Three-Phase Series RLC Load ==
  Electrical Reference : fl_lib/Electrical/Electrical Elements/Electrical Reference
  Wye-Connected Load : ee_lib/Passive/RLC Assemblies/Wye-Connected Load  port_option=ee.enum.threePhasePort.expanded  parameterization=2  component_structure=7  component_structure_PQ=7  R=1 Ohm  L=0.001 H  C=1e-6 F  VRated=1000 V  FRated=60 Hz  P=10000 W  Qpos=100 V*A  Qneg=Three_PhaseSeriesRLCLoad_class(100).objParamMappingDerived.NewDerivedParam.Qneg V*A  R_parasitic=1e-6 Ohm  G_parasitic=1e-6 1/Ohm  R_parasitic_PQ=1e-6 Ohm  G_parasitic_PQ=1e-6 1/Ohm  Vmag0=1000 V  Vang0=0 deg  Freq0=60 Hz  IL_specify=on  IL_priority=High  IL=[ 0 0 0 ] A  IL_nominal_specify=off  IL_nominal_value=1  IL_nominal_unit=A  VC_specify=on  VC_priority=High  VC=[ 0 0 0 ] V  VC_nominal_specify=off  VC_nominal_value=1  VC_nominal_unit=V
      settings: InternalSimscapePortConfiguration="{\"Bottom\":[],\"Left\":[{\"id\":\"a\",\"label\":\"a\",\"type\":\"foundation.electrical.electrical\"},{\"id\":\"b\",\"label\":\"b\",\"type\":\"foundation.electrical.electrical\"},{\"id\":\"c\",\"label\":\"c\",\"type\":\"foundation.electrical.electrical\"}],\"Right\":[{\"id\":\"n\",\"label\":\"n\",\"type\":\"foundation.electrical.electrical\"}],\"Top\":[]}"
  A : PMIOPort  Side=Left
  B : PMIOPort  Port=2  Side=Left
  C : PMIOPort  Port=3  Side=Left
  connections:
  Electrical Reference/LConn1 -- Wye-Connected Load/RConn1
  Wye-Connected Load/LConn3 -- C/RConn1
  Wye-Connected Load/LConn1 -- A/RConn1
  Wye-Connected Load/LConn2 -- B/RConn1

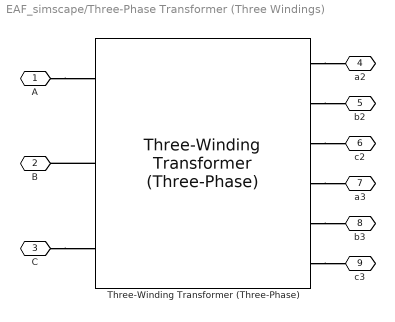
== system EAF_simscape/Three-Phase Transformer (Three Windings) ==
  Three-Winding Transformer (Three-Phase) : ee_lib/Passive/Transformers/Three-Winding Transformer (Three-Phase)  SRated=250000000 V*A  FRated=60 Hz  Winding1Connection=3  VRated1=110000 V  Winding2Connection=3  VRated2=35000 V  Winding3Connection=3  VRated3=35000 V  CoreType=2  pu_Rw1=Three_PhaseTransformer_T_class('Yg','Yg','Yg','pu',[250000000 60],[110000 1.186 0.08],[35000 0.256 0.08],[35000 0.002 0.08],499.98,500,0.5,[0 0;0.0024 1.2;1 1.52],[0.8 -0.8 0.69999],'off','off').objParamMappingDerived.NewDerivedParam.pu_Rw1  pu_Rw2=Three_PhaseTransformer_T_class('Yg','Yg','Yg','pu',[250000000 60],[110000 1.186 0.08],[35000 0.256 0.08],[35000 0.002 0.08],499.98,500,0.5,[0 0;0.0024 1.2;1 1.52],[0.8 -0.8 0.69999],'off','off').objParamMappingDerived.NewDerivedParam.pu_Rw2  pu_Rw3=Three_PhaseTransformer_T_class('Yg','Yg','Yg','pu',[250000000 60],[110000 1.186 0.08],[35000 0.256 0.08],[35000 0.002 0.08],499.98,500,0.5,[0 0;0.0024 1.2;1 1.52],[0.8 -0.8 0.69999],'off','off').objParamMappingDerived.NewDerivedParam.pu_Rw3  leakage_reactance_option=ee.enum.transformer_leakage.include  pu_Xl1=Three_PhaseTransformer_T_class('Yg','Yg','Yg','pu',[250000000 60],[110000 1.186 0.08],[35000 0.256 0.08],[35000 0.002 0.08],499.98,500,0.5,[0 0;0.0024 1.2;1 1.52],[0.8 -0.8 0.69999],'off','off').objParamMappingDerived.NewDerivedParam.pu_Xl1  pu_Xl2=Three_PhaseTransformer_T_class('Yg','Yg','Yg','pu',[250000000 60],[110000 1.186 0.08],[35000 0.256 0.08],[35000 0.002 0.08],499.98,500,0.5,[0 0;0.0024 1.2;1 1.52],[0.8 -0.8 0.69999],'off','off').objParamMappingDerived.NewDerivedParam.pu_Xl2  pu_Xl3=Three_PhaseTransformer_T_class('Yg','Yg','Yg','pu',[250000000 60],[110000 1.186 0.08],[35000 0.256 0.08],[35000 0.002 0.08],499.98,500,0.5,[0 0;0.0024 1.2;1 1.52],[0.8 -0.8 0.69999],'off','off').objParamMappingDerived.NewDerivedParam.pu_Xl3  magnetizing_resistance_option=ee.enum.transformer_magnetizingResistance.include  pu_Rm=Three_PhaseTransformer_T_class('Yg','Yg','Yg','pu',[250000000 60],[110000 1.186 0.08],[35000 0.256 0.08],[35000 0.002 0.08],499.98,500,0.5,[0 0;0.0024 1.2;1 1.52],[0.8 -0.8 0.69999],'off','off').objParamMappingDerived.NewDerivedParam.pu_Rm  magnetizing_reactance_option=ee.enum.transformer_magnetizingReactance.include  saturation_option=1  pu_Xm=Three_PhaseTransformer_T_class('Yg','Yg','Yg','pu',[250000000 60],[110000 1.186 0.08],[35000 0.256 0.08],[35000 0.002 0.08],499.98,500,0.5,[0 0;0.0024 1.2;1 1.52],[0.8 -0.8 0.69999],'off','off').objParamMappingDerived.NewDerivedParam.pu_Xm  current_data=Three_PhaseTransformer_T_class('Yg','Yg','Yg','pu',[250000000 60],[110000 1.186 0.08],[35000 0.256 0.08],[35000 0.002 0.08],499.98,500,0.5,[0 0;0.0024 1.2;1 1.52],[0.8 -0.8 0.69999],'off','off').objParamMappingDerived.NewDerivedParam.current_data  magnetic_flux_data=Three_PhaseTransformer_T_class('Yg','Yg','Yg','pu',[250000000 60],[110000 1.186 0.08],[35000 0.256 0.08],[35000 0.002 0.08],499.98,500,0.5,[0 0;0.0024 1.2;1 1.52],[0.8 -0.8 0.69999],'off','off').objParamMappingDerived.NewDerivedParam.magnetic_flux_data  pu_X0=Three_PhaseTransformer_T_class('Yg','Yg','Yg','pu',[250000000 60],[110000 1.186 0.08],[35000 0.256 0.08],[35000 0.002 0.08],499.98,500,0.5,[0 0;0.0024 1.2;1 1.52],[0.8 -0.8 0.69999],'off','off').objParamMappingDerived.NewDerivedParam.pu_X0  i1_specify=off  i1_priority=None  i1=[ 0 0 0 ] A  i1_nominal_specify=off  i1_nominal_value=1  i1_nominal_unit=A  i2_specify=off  i2_priority=None  i2=[ 0 0 0 ] A  i2_nominal_specify=off  i2_nominal_value=1  i2_nominal_unit=A  i3_specify=off  i3_priority=None  i3=[ 0 0 0 ] A  i3_nominal_specify=off  i3_nominal_value=1  i3_nominal_unit=A  phi_specify=off  phi_priority=None  phi=Three_PhaseTransformer_T_class('Yg','Yg','Yg','pu',[250000000 60],[110000 1.186 0.08],[35000 0.256 0.08],[35000 0.002 0.08],499.98,500,0.5,[0 0;0.0024 1.2;1 1.52],[0.8 -0.8 0.69999],'off','off').objParamMappingDerived.NewDerivedParam.phi  phi_nominal_specify=off  phi_nominal_value=1  phi_nominal_unit=1  power_dissipated_specify=off  power_dissipated_priority=None  power_dissipated=0 W  power_dissipated_nominal_specify=off  power_dissipated_nominal_value=1  power_dissipated_nominal_unit=W
      settings: InternalSimscapePortConfiguration="{\"Bottom\":[],\"Left\":[{\"id\":\"a1\",\"label\":\"a1\",\"type\":\"foundation.electrical.electrical\"},{\"id\":\"b1\",\"label\":\"b1\",\"type\":\"foundation.electrical.electrical\"},{\"id\":\"c1\",\"label\":\"c1\",\"type\":\"foundation.electrical.electrical\"}],\"Right\":[{\"id\":\"a2\",\"label\":\"a2\",\"type\":\"foundation.electrical.electrical\"},{\"id\":\"b2\",\"label\":\"b2\",\"type\":\"foundation.electrical.electrical\"},{\"id\":\"c2\",\"label\":\"c2\",\"type\":\"foundation.electrical.electrical\"},{\"id\":\"a3\",\"label\":\"a3\",\"type\":\"foundation.electrical.electrical\"},{\"id\":\"b3\",\"label\":\"b3\",\"type\":\"foundation.electrical.electrical\"},{\"id\":\"c3\",\"label\":\"c3\",\"type\":\"foundation.electrical.electrical\"}],\"Top\":[]}"
  A : PMIOPort  Side=Left
  B : PMIOPort  Port=2  Side=Left
  C : PMIOPort  Port=3  Side=Left
  a2 : PMIOPort  Port=4  Side=Right
  b2 : PMIOPort  Port=5  Side=Right
  c2 : PMIOPort  Port=6  Side=Right
  a3 : PMIOPort  Port=7  Side=Right
  b3 : PMIOPort  Port=8  Side=Right
  c3 : PMIOPort  Port=9  Side=Right
  connections:
  Three-Winding Transformer (Three-Phase)/RConn3 -- c2/RConn1
  Three-Winding Transformer (Three-Phase)/RConn2 -- b2/RConn1
  Three-Winding Transformer (Three-Phase)/RConn1 -- a2/RConn1
  A/RConn1 -- Three-Winding Transformer (Three-Phase)/LConn1
  Three-Winding Transformer (Three-Phase)/LConn2 -- B/RConn1
  C/RConn1 -- Three-Winding Transformer (Three-Phase)/LConn3
  Three-Winding Transformer (Three-Phase)/RConn4 -- a3/RConn1
  Three-Winding Transformer (Three-Phase)/RConn5 -- b3/RConn1
  Three-Winding Transformer (Three-Phase)/RConn6 -- c3/RConn1
